simulink model "SmartTrafficControl_Simulation"  (R2024b)
settings: Solver=VariableStepAuto  StartTime=0.0  StopTime=10.0  RelTol=1e-3
(part 2 of 2)

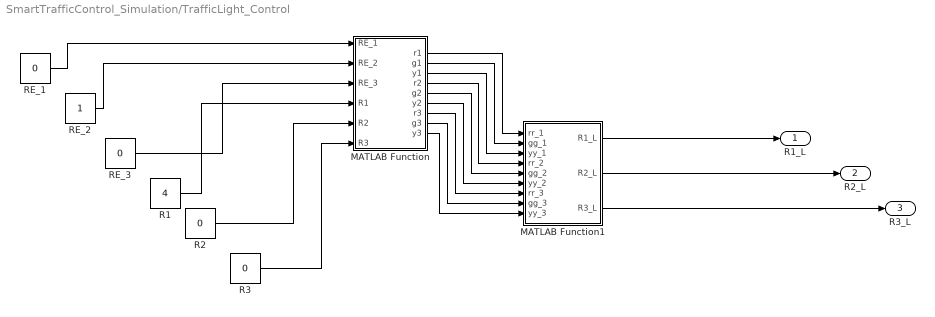
== system SmartTrafficControl_Simulation/TrafficLight_Control ==
  MATLAB Function : MATLAB Function  TreatAsAtomicUnit=on
  MATLAB Function1 : MATLAB Function  TreatAsAtomicUnit=on
  R1 : Constant  Value=4
  R2 : Constant  Value=0
  R3 : Constant  Value=0
  RE_1 : Constant  Value=0
  RE_2 : Constant
  RE_3 : Constant  Value=0
  R1_L : Outport
  R2_L : Outport  Port=2
  R3_L : Outport  Port=3
  wires:
  R1/1 -> MATLAB Function/4(R1)
  MATLAB Function1/3(R3_L) -> R3_L/1
  MATLAB Function/3(y1) -> MATLAB Function1/3(yy_1)
  MATLAB Function/9(y3) -> MATLAB Function1/9(yy_3)
  RE_1/1 -> MATLAB Function/1(RE_1)
  MATLAB Function/6(y2) -> MATLAB Function1/6(yy_2)
  R3/1 -> MATLAB Function/6(R3)
  MATLAB Function/5(g2) -> MATLAB Function1/5(gg_2)
  MATLAB Function/7(r3) -> MATLAB Function1/7(rr_3)
  R2/1 -> MATLAB Function/5(R2)
  MATLAB Function1/2(R2_L) -> R2_L/1
  MATLAB Function/2(g1) -> MATLAB Function1/2(gg_1)
  MATLAB Function/1(r1) -> MATLAB Function1/1(rr_1)
  MATLAB Function/4(r2) -> MATLAB Function1/4(rr_2)
  MATLAB Function/8(g3) -> MATLAB Function1/8(gg_3)
  MATLAB Function1/1(R1_L) -> R1_L/1
  RE_2/1 -> MATLAB Function/2(RE_2)
  RE_3/1 -> MATLAB Function/3(RE_3)

== matlab function SmartTrafficControl_Simulation/TrafficLight_Control/MATLAB Function1 ==
  data: rr_1 input; R1_L output; gg_1 input; yy_1 input; R2_L output; R3_L output; rr_2 input; gg_2 input; yy_2 input; rr_3 input; gg_3 input; yy_3 input
function [R1_L,R2_L,R3_L] = lightcontrol(rr_1,gg_1,yy_1,rr_2,gg_2,yy_2,rr_3,gg_3,yy_3)


  if  gg_1 ==1
      R1_L =1;
      R2_L =2;
      R3_L = 3;
  elseif gg_2 ==1
      R2_L =1;
      R3_L =2;
      R1_L =3;
  else

      R2_L =3;
      R3_L =1;
      R1_L =2;

end

== matlab function SmartTrafficControl_Simulation/TrafficLight_Control/MATLAB Function ==
  data: RE_1 input; r1 output; RE_2 input; RE_3 input; R1 input; R2 input; R3 input; g1 output; y1 output; r2 output; g2 output; y2 output; r3 output; g3 output; y3 output
function [r1,g1,y1,r2,g2,y2,r3,g3,y3] = Smartraffic(RE_1,RE_2,RE_3,R1,R2,R3)

    r1 =0 ,g1 =0, y1= 0;
    r2 =0 ,g2 = 0, y2 =0;
    r3 =0, g3 =0 ,y3 =0;



if R1 >R2 & R1>R3
    r1 =0, g1 =1, y1= 0;
    r2 =0, g2 = 0, y2 =1;
    r3 =1, g3 =0, y3 =0;
elseif R2 > R3
    r1 =1, g1 =0, y1= 0;
    r2 =0, g2 = 1, y2 =0;
    r3 =0, g3 =0, y3 =1;
elseif R3 > R2 & R3 > R1
    r1 =0, g1 =0, y1= 1;
    r2 =1, g2 = 0, y2 =0;
    r3 =0, g3 =1, y3 =0;
end
if RE_1 == 1
    r1 =0 ,g1 =1, y1= 0;
    r2 =0 ,g2 = 0, y2 =1;
    r3 =1, g3 =0 ,y3 =0;
elseif RE_2 ==1
    r1 =1, g1 =0, y1= 0;
    r2 =0, g2 = 1, y2 =0;
    r3 =0, g3 =0, y3 =1;
elseif RE_3 ==1
    r1 =0, g1 =0, y1= 1;
    r2 =1, g2 = 0, y2 =0;
    r3 =0, g3 =1, y3 =0;
end





end
